simulink model "template_CR1_PreRTHS"  (Simulink 8.2)
settings: Solver=FixedStepDiscrete  StartTime=0.0  StopTime=RunningTime  FixedStep=sample  RelTol=1e-3
undefined symbols (not defined in the file): ElementsStruct, Integrator, NumFreeDOF, RigidLinkMasterMatrix, RigidLinkNo, RigidLinkNodeID, RigidLinkSlaveMatrix, sample, SampleRate, Structure
libraries: HybridFEMLibrary x2
(part 1 of 2)
CloseFcn:
  | rtwprivate ssgencode ModelCloseRequest hybriddaq1dof
settings Model: MinMaxOverflowLogging=ForceOff  Creator=RTMD  LastModifiedBy=Thomas Marullo  BufferReuse=off
settings DataIOCC: LimitDataPoints=off
settings OptimizationCC: BlockReduction=off  OptimizeBlockIOStorage=off  BufferReuse=off  ExpressionFolding=off  LocalBlockOutputs=off  InitFltsAndDblsToZero=on
settings DebuggingCC: SignalResolutionControl=TryResolveAllWithWarning  MultiTaskDSMMsg=warning  FcnCallInpInsideContextMsg=EnableAllAsWarning
settings HardwareCC: ProdIntDivRoundTo=Zero  ProdEndianess=LittleEndian  ProdHWDeviceType=Generic->32-bit x86 compatible
settings SFSimCC: SimParseCustomCode=off
settings RTWCC: ProcessScript=grt_make_rtw_hook  RTWCompilerOptimization=On
settings GRTTargetCC: CombineOutputUpdateFcns=on  GRTInterface=off

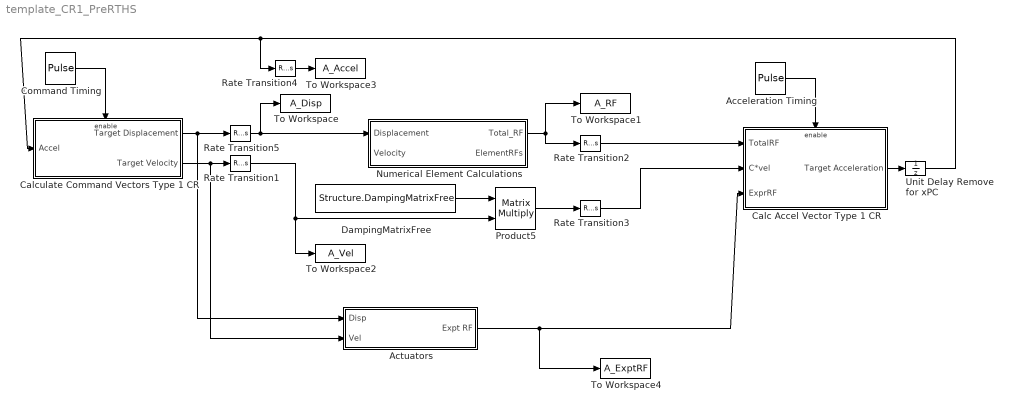
== system template_CR1_PreRTHS ==
  Acceleration Timing : DiscretePulseGenerator  Period=Integrator.Interpolations  PhaseDelay=Integrator.Interpolations-1  SampleTime=sample
  Actuators : Subsystem
  Calc Accel Vector Type 1 CR : Subsystem
  Calculate Command Vectors Type 1 CR : Subsystem  TreatAsAtomicUnit=on  SystemSampleTime=SampleRate
  Command Timing : DiscretePulseGenerator  Period=Integrator.Interpolations  SampleTime=sample
  DampingMatrixFree : Constant  Value=Structure.DampingMatrixFree
  Numerical Element Calculations : MATLAB Function  TreatAsAtomicUnit=on
  Product5 : Product  Multiplication=Matrix(*)  RndMeth=Zero
  Rate Transition1 : RateTransition  Deterministic=off  OutPortSampleTime=SampleRate
  Rate Transition2 : RateTransition  Deterministic=off  OutPortSampleTime=sample
  Rate Transition3 : RateTransition  Deterministic=off  OutPortSampleTime=sample
  Rate Transition4 : RateTransition  Deterministic=off  OutPortSampleTime=SampleRate
  Rate Transition5 : RateTransition  Deterministic=off  OutPortSampleTime=SampleRate
  To Workspace : ToWorkspace  VariableName=A_Disp  SampleTime=-1
  To Workspace1 : ToWorkspace  VariableName=A_RF  SampleTime=-1
  To Workspace2 : ToWorkspace  VariableName=A_Vel  SampleTime=-1
  To Workspace3 : ToWorkspace  VariableName=A_Accel  SampleTime=-1
  To Workspace4 : ToWorkspace  VariableName=A_ExptRF  SampleTime=-1
  Unit Delay Remove for xPC : UnitDelay  SampleTime=-1
  wires:
  Acceleration Timing/1 -> Calc Accel Vector Type 1 CR/Enable
  Calc Accel Vector Type 1 CR/1(Target Acceleration) -> Unit Delay Remove for xPC/1
  Numerical Element Calculations/1(Total_RF) -> Rate Transition2/1, To Workspace1/1
  Rate Transition2/1 -> Calc Accel Vector Type 1 CR/1(TotalRF)
  Command Timing/1 -> Calculate Command Vectors Type 1 CR/Enable
  Calculate Command Vectors Type 1 CR/1(Target Displacement) -> Actuators/1(Disp), Rate Transition5/1
  Rate Transition5/1 -> Numerical Element Calculations/1(Displacement), To Workspace/1
  Unit Delay Remove for xPC/1 -> Rate Transition4/1, Calculate Command Vectors Type 1 CR/1(Accel)
  DampingMatrixFree/1 -> Product5/1
  Product5/1 -> Rate Transition3/1
  Rate Transition1/1 -> Product5/2, To Workspace2/1
  Rate Transition3/1 -> Calc Accel Vector Type 1 CR/2(C*vel)
  Rate Transition4/1 -> To Workspace3/1
  Calculate Command Vectors Type 1 CR/2(Target Velocity) -> Actuators/2(Vel), Rate Transition1/1
  Actuators/1(Expt RF) -> To Workspace4/1, Calc Accel Vector Type 1 CR/3(ExprRF)

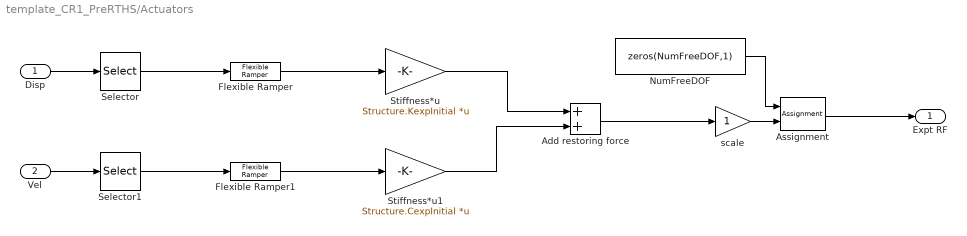
== system template_CR1_PreRTHS/Actuators ==
  Disp : Inport
  Vel : Inport  Port=2
  Add restoring force : Sum
  Assignment : Assignment  IndexOptions=Index vector (dialog)  Indices=Structure.InterfaceDOF  OutputSizes=1
  Flexible Ramper : HybridFEMLibrary/Flexible Ramper  ramps=Integrator.Interpolations  samplerate=sample  initVal=zeros(size(Structure.InterfaceDOF),1)
  Flexible Ramper1 : HybridFEMLibrary/Flexible Ramper  ramps=Integrator.Interpolations  samplerate=sample  initVal=zeros(size(Structure.InterfaceDOF),1)
  NumFreeDOF : Constant  Value=zeros(NumFreeDOF,1)
  Selector : Selector  InputPortWidth=NumFreeDOF  IndexOptions=Index vector (dialog)  Indices=Structure.InterfaceDOF  OutputSizes=1
  Selector1 : Selector  InputPortWidth=NumFreeDOF  IndexOptions=Index vector (dialog)  Indices=Structure.InterfaceDOF  OutputSizes=1
  Stiffness*u : Gain  Gain=Structure.KexpInitial  Multiplication=Matrix(K*u) (u vector)
  Stiffness*u1 : Gain  Gain=Structure.CexpInitial  Multiplication=Matrix(K*u) (u vector)
  scale : Gain
  Expt RF : Outport
  wires:
  Disp/1 -> Selector/1
  Vel/1 -> Selector1/1
  Selector/1 -> Flexible Ramper/1
  Selector1/1 -> Flexible Ramper1/1
  Assignment/1 -> Expt RF/1
  Stiffness*u/1 -> Add restoring force/1
  Add restoring force/1 -> scale/1
  NumFreeDOF/1 -> Assignment/1
  scale/1 -> Assignment/2
  Stiffness*u1/1 -> Add restoring force/2
  Flexible Ramper/1 -> Stiffness*u/1
  Flexible Ramper1/1 -> Stiffness*u1/1

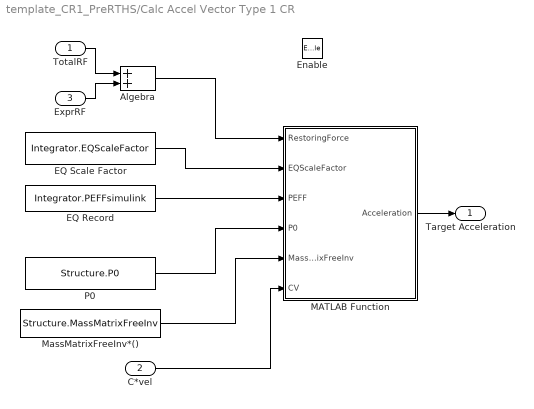
== system template_CR1_PreRTHS/Calc Accel Vector Type 1 CR ==
  TotalRF : Inport
  C*vel : Inport  Port=2
  ExprRF : Inport  Port=3
  Enable : EnablePort
  Algebra : Sum
  EQ Record : FromWorkspace  VariableName=Integrator.PEFFsimulink  Interpolate=off  OutputAfterFinalValue=Setting to zero
  EQ Scale Factor : Constant  Value=Integrator.EQScaleFactor
  MATLAB Function : MATLAB Function  TreatAsAtomicUnit=on
  MassMatrixFreeInv*() : Constant  Value=Structure.MassMatrixFreeInv
  P0 : Constant  Value=Structure.P0
  Target Acceleration : Outport
  wires:
  MATLAB Function/1(Acceleration) -> Target Acceleration/1
  TotalRF/1 -> Algebra/1
  ExprRF/1 -> Algebra/2
  Algebra/1 -> MATLAB Function/1(RestoringForce)
  EQ Scale Factor/1 -> MATLAB Function/2(EQScaleFactor)
  EQ Record/1 -> MATLAB Function/3(PEFF)
  P0/1 -> MATLAB Function/4(P0)
  MassMatrixFreeInv*()/1 -> MATLAB Function/5(MassMatrixFreeInv)
  C*vel/1 -> MATLAB Function/6(CV)

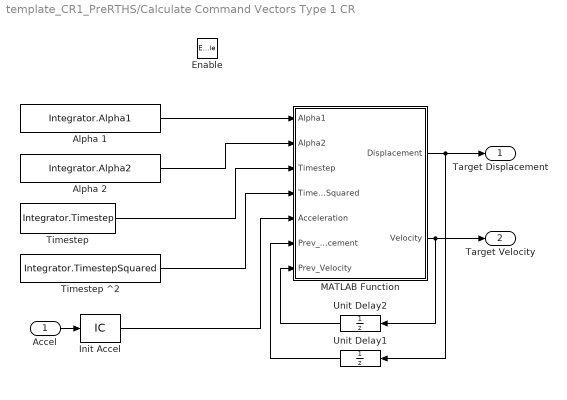
== system template_CR1_PreRTHS/Calculate Command Vectors Type 1 CR ==
  Accel : Inport
  Enable : EnablePort
  Alpha 1 : Constant  Priority=5  Value=Integrator.Alpha1
  Alpha 2 : Constant  Priority=11  Value=Integrator.Alpha2
  Init Accel : InitialCondition  Priority=2  Value=Integrator.Acceleration
  MATLAB Function : MATLAB Function  TreatAsAtomicUnit=on
  "Timestep " : Constant  Priority=3  Value=Integrator.Timestep
  Timestep ^2 : Constant  Priority=9  Value=Integrator.TimestepSquared
  Unit Delay1 : UnitDelay  Priority=7  SampleTime=-1
  Unit Delay2 : UnitDelay  Priority=7  SampleTime=-1
  Target Displacement : Outport
  Target Velocity : Outport  Port=2
  wires:
  Accel/1 -> Init Accel/1
  MATLAB Function/1(Displacement) -> Target Displacement/1, Unit Delay1/1
  MATLAB Function/2(Velocity) -> Target Velocity/1, Unit Delay2/1
  Unit Delay1/1 -> MATLAB Function/6(Prev_Displacement)
  Unit Delay2/1 -> MATLAB Function/7(Prev_Velocity)
  Alpha 1/1 -> MATLAB Function/1(Alpha1)
  Alpha 2/1 -> MATLAB Function/2(Alpha2)
  "Timestep "/1 -> MATLAB Function/3(Timestep)
  Timestep ^2/1 -> MATLAB Function/4(TimestepSquared)
  Init Accel/1 -> MATLAB Function/5(Acceleration)

== matlab function Calc Accel Vector Type 1 CR/MATLAB Function ==
  data: RestoringForce input double; EQScaleFactor input double; PEFF input double; P0 input double; MassMatrixFreeInv input double; Acceleration output double; CV input double
function Acceleration  = fcn(RestoringForce,...                              
                            EQScaleFactor,...
                            PEFF,...      
                            P0,... 
                            MassMatrixFreeInv,...
                            CV...
                            )
                                                
Acceleration = MassMatrixFreeInv * ...
                  (EQScaleFactor * PEFF - CV ...
                   - RestoringForce + P0);
